simulink model "model_v420"  (R2020a)
settings: Solver=VariableStepAuto  StartTime=0.0  StopTime=200  RelTol=1e-3
settings Model: Creator=Piotr  LastModifiedBy=Piotr

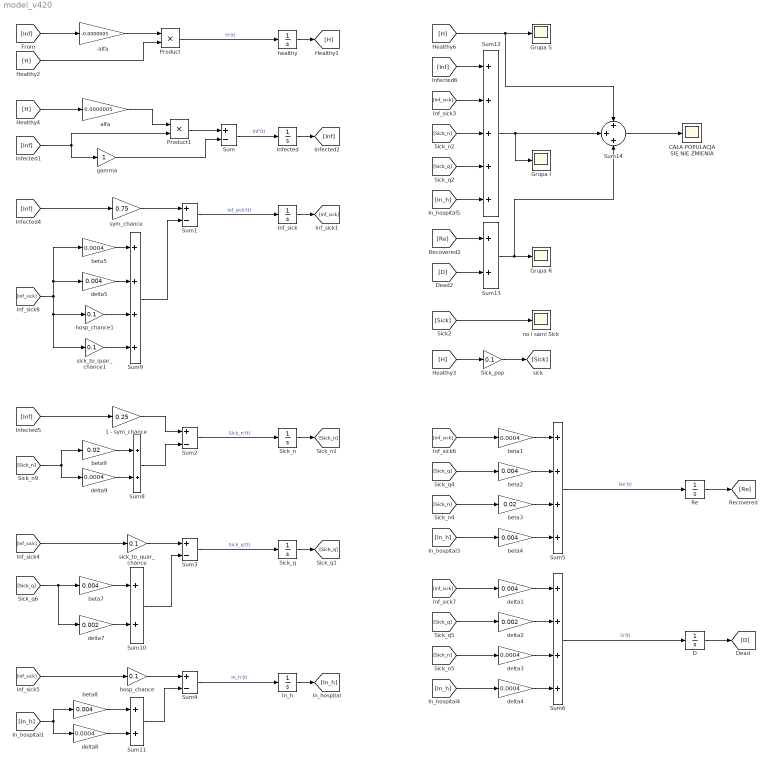
== system model_v420 ==
  -alfa : Gain  Gain=-0.0000005
  1 - sym_chance : Gain  Gain=0.25
  CAŁA POPULACJA SIĘ NIE ZMIENIA : Scope
  D : Integrator
  Grupa I : Scope
  Grupa R : Scope
  Grupa S : Scope
  In_h : Integrator
  Inf_sick : Integrator
  Infected : Integrator  InitialCondition=1
  Product : Product
  Product1 : Product
  Re : Integrator
  Sick_n : Integrator
  Sick_pop : Gain  Gain=0.1
  Sick_q : Integrator
  Sum{,1..4} (5 alike) : Sum  Inputs=+-
  Sum{8,10..11,13} (4 alike) : Sum
  Sum12 : Sum  Inputs=+++++
  Sum14 : Sum  Inputs=+++
  Sum5 : Sum  Inputs=++++
  Sum6 : Sum  Inputs=++++
  Sum9 : Sum  Inputs=++++
  alfa : Gain  Gain=0.0000005
  beta1 : Gain  Gain=0.0004
  beta{2,4,7..8} (4 alike) : Gain  Gain=0.004
  beta3 : Gain  Gain=0.02
  beta5 : Gain  Gain=0.0004
  beta9 : Gain  Gain=0.02
  delta1 : Gain  Gain=0.004
  delta2 : Gain  Gain=0.002
  delta{3..4,8..9} (4 alike) : Gain  Gain=0.0004
  delta5 : Gain  Gain=0.004
  delta7 : Gain  Gain=0.002
  gamma : Gain
  healthy : Integrator  InitialCondition=3000000
  hosp_chance : Gain  Gain=0.1
  hosp_chance1 : Gain  Gain=0.1
  no i sami Sick : Scope
  sick_to_quar_chance : Gain  Gain=0.1
  sick_to_quar_chance1 : Gain  Gain=0.1
  sym_chance : Gain  Gain=0.75
  wires:
  healthy/1 -> [H]
  -alfa/1 -> Product/1
  [Inf] -> -alfa/1
  Product/1 -> healthy/1  "H'(t)"
  [H] -> Product/2
  [H] -> Sick_pop/1
  Sick_pop/1 -> [Sick]
  Sum/1 -> Infected/1  "Inf'(t)"
  [Inf] -> gamma/1, Product1/2
  gamma/1 -> Sum/2
  [H] -> alfa/1
  alfa/1 -> Product1/1
  Product1/1 -> Sum/1
  Infected/1 -> [Inf]
  [Inf] -> sym_chance/1
  sym_chance/1 -> Sum1/1
  Sum1/1 -> Inf_sick/1  "Inf_sick'(t)"
  Inf_sick/1 -> [Inf_sick]
  Sum2/1 -> Sick_n/1  "Sick_n'(t)"
  Sick_n/1 -> [Sick_n]
  1 - sym_chance/1 -> Sum2/1
  [Inf] -> 1 - sym_chance/1
  Sum3/1 -> Sick_q/1  "Sick_q'(t)"
  Sick_q/1 -> [Sick_q]
  sick_to_quar_chance/1 -> Sum3/1
  Sum4/1 -> In_h/1  "In_h'(t)"
  In_h/1 -> [In_h]
  hosp_chance/1 -> Sum4/1
  beta2/1 -> Sum5/2
  beta1/1 -> Sum5/1
  beta3/1 -> Sum5/3
  Sum5/1 -> Re/1  "Re'(t)"
  Re/1 -> [Re]
  beta4/1 -> Sum5/4
  delta2/1 -> Sum6/2
  delta4/1 -> Sum6/4
  Sum6/1 -> D/1  "D'(t)"
  delta3/1 -> Sum6/3
  delta1/1 -> Sum6/1
  D/1 -> [D]
  [Inf_sick] -> beta5/1, delta5/1, hosp_chance1/1, sick_to_quar_chance1/1
  [Inf_sick] -> beta1/1
  [Sick_q] -> beta2/1
  [Sick_n] -> beta3/1
  [Inf_sick] -> delta1/1
  [Sick_q] -> delta2/1
  [Sick_n] -> delta3/1
  [In_h] -> delta4/1
  [Inf_sick] -> hosp_chance/1
  [Sick_q] -> beta7/1, delta7/1
  [Inf_sick] -> sick_to_quar_chance/1
  [In_h] -> beta4/1
  [In_h] -> beta8/1, delta8/1
  [Sick_n] -> delta9/1, beta9/1
  beta9/1 -> Sum8/1
  delta9/1 -> Sum8/2
  Sum8/1 -> Sum2/2
  beta5/1 -> Sum9/1
  delta5/1 -> Sum9/2
  hosp_chance1/1 -> Sum9/3
  sick_to_quar_chance1/1 -> Sum9/4
  Sum9/1 -> Sum1/2
  beta7/1 -> Sum10/1
  delta7/1 -> Sum10/2
  Sum10/1 -> Sum3/2
  beta8/1 -> Sum11/1
  delta8/1 -> Sum11/2
  Sum11/1 -> Sum4/2
  [H] -> Sum14/1, Grupa S/1
  [Inf] -> Sum12/1
  [Inf_sick] -> Sum12/2
  [Sick_n] -> Sum12/3
  [Sick_q] -> Sum12/4
  [In_h] -> Sum12/5
  Sum12/1 -> Sum14/2, Grupa I/1
  [Re] -> Sum13/1
  [D] -> Sum13/2
  Sum13/1 -> Sum14/3, Grupa R/1
  Sum14/1 -> CAŁA POPULACJA SIĘ NIE ZMIENIA/1
  [Sick] -> no i sami Sick/1
